simulink library "sample_model"  (Simulink 8.6)
settings: Solver=ode45  StartTime=0.0  StopTime=10.0  RelTol=1e-3
undefined symbols (not defined in the file): K_FOO_BAR
settings Model: Creator=q284114  LastModifiedBy=q284114

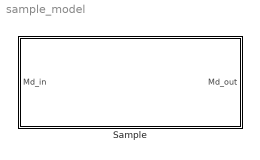
== system sample_model ==
  Sample : Subsystem

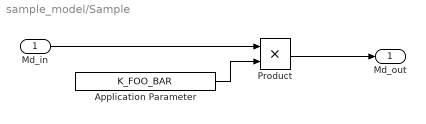
== system sample_model/Sample ==
  Md_in : Inport
  Application Parameter : Constant  Value=K_FOO_BAR
      settings: AttributesFormatString=%<Value>
  Product : Product  OutDataTypeStr=Inherit: Inherit via back propagation  RndMeth=Simplest  SaturateOnIntegerOverflow=on
  Md_out : Outport
  wires:
  Md_in/1 -> Product/1
  Application Parameter/1 -> Product/2
  Product/1 -> Md_out/1
